simulink model "linear_vehicle_model"  (R2018a)
settings: Solver=VariableStepAuto  StartTime=0.0  StopTime=450  RelTol=1e-3
values from neighbouring files (symbols this model uses):
  Err_matrix = [1 -1 0 0 0 0 ... (first row only)    [Simulation_variables.m]
  vel_pos = [1 0 0]    [Simulation_variables.m]
  vel_vet = [0 1 0]    [Simulation_variables.m]
undefined symbols (not defined in the file or in its folder): controller, Reference, Vehicle, vehicleL
settings Model: Creator=um0002  LastModifiedBy=mw00361
settings SFSimCC: SimUseLocalCustomCode=on
settings RTWCC: RTWUseLocalCustomCode=on

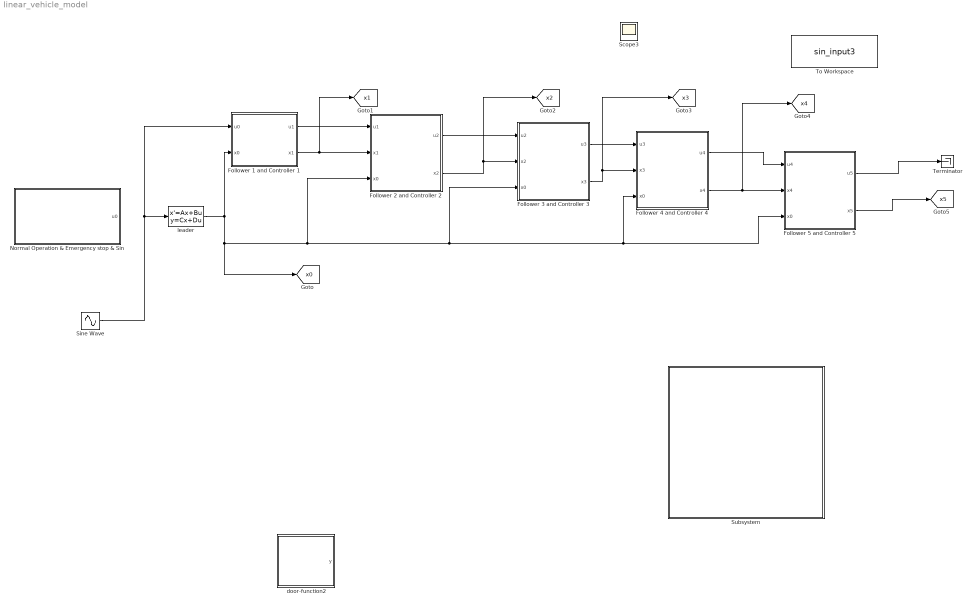
== system linear_vehicle_model ==
  Follower 1 and Controller 1 : Subsystem
  Follower 2 and Controller 2 : Subsystem
  Follower 3 and Controller 3 : Subsystem
  Follower 4 and Controller 4 : Subsystem
  Follower 5 and Controller 5 : Subsystem
  Normal Operation & Emergency stop & Sin : Subsystem
  Scope3 : Scope
  Sine Wave : Sin  Amplitude=200  Frequency=3  SampleTime=0
  Subsystem : Subsystem
  Terminator : Terminator
  To Workspace : ToWorkspace  VariableName=sin_input3  SaveFormat=Timeseries  SampleTime=-1
  door-function2 : Subsystem  mask{t_start=150, t_end=152, H=1.5}
      mask prompts: t_start "initial time"; t_end "final time"; H "height"
  leader : StateSpace  A=[0 1 0; 0 0 1; 0 0 -1/vehicleL.tau]  B=[0 0 1/vehicleL.tau]'  C=eye(3)  D=zeros(3,1)  InitialCondition=[100 75/3.6 0]'
  tag scope: x0=global, x1=global, x2=global, x3=global, x4=global, x5=global
  wires:
  Follower 1 and Controller 1/1("u1 ") -> Follower 2 and Controller 2/1(u1)
  Follower 1 and Controller 1/2(x1) -> [x1], Follower 2 and Controller 2/2(x1)
  Follower 2 and Controller 2/1("u2 ") -> Follower 3 and Controller 3/1(u2)
  Follower 3 and Controller 3/1("u3 ") -> Follower 4 and Controller 4/1(u3)
  Follower 3 and Controller 3/2(x3) -> [x3], Follower 4 and Controller 4/2(x3)
  Follower 2 and Controller 2/2(x2) -> [x2], Follower 3 and Controller 3/2(x2)
  leader/1 -> [x0], Follower 2 and Controller 2/3("x0 "), Follower 3 and Controller 3/3("x0 "), Follower 5 and Controller 5/3("x0 "), Follower 4 and Controller 4/3("x0 "), Follower 1 and Controller 1/2(x0)
  Follower 4 and Controller 4/1("u4 ") -> Follower 5 and Controller 5/1(u4)
  Follower 4 and Controller 4/2(x4) -> Follower 5 and Controller 5/2(x4), [x4]
  Follower 5 and Controller 5/1("u5 ") -> Terminator/1
  Follower 5 and Controller 5/2(x5) -> [x5]
  Sine Wave/1 -> Follower 1 and Controller 1/1(u0), leader/1

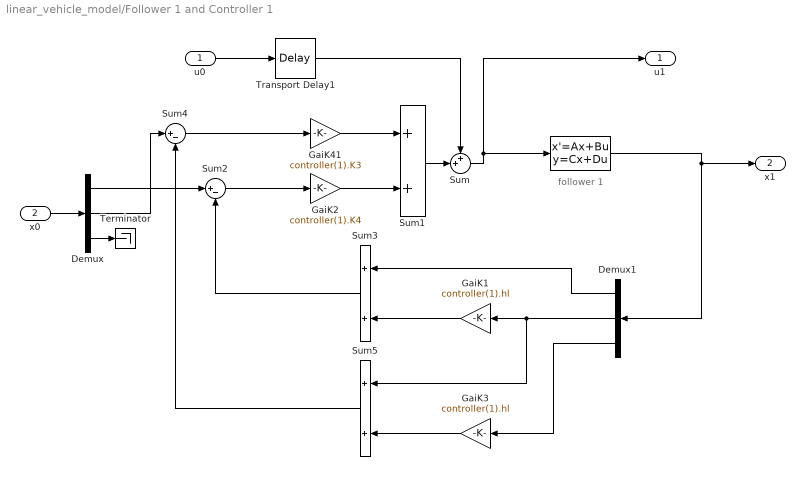
== system linear_vehicle_model/Follower 1 and Controller 1 ==
  note: follower 1
  u0 : Inport
  x0 : Inport  Port=2
  " " : StateSpace  A=[0 1 0; 0 0 1; 0 0 -1/vehicleL.tau]  B=[0 0 1/Vehicle(1).tau]'  C=eye(3)  D=zeros(3,1)  InitialCondition=[Vehicle(1).s0 75/3.6 0]'
  Demux : Demux  Outputs=3
  Demux1 : Demux  Outputs=3
  GaiK1 : Gain  Gain=controller(1).hl
  GaiK2 : Gain  Gain=controller(1).K4
  GaiK3 : Gain  Gain=controller(1).hl
  GaiK41 : Gain  Gain=controller(1).K3
  Sum : Sum  Inputs=++|
  Sum1 : Sum
  Sum2 : Sum  Inputs=|+-
  Sum3 : Sum
  Sum4 : Sum  Inputs=|+-
  Sum5 : Sum
  Terminator : Terminator
  Transport Delay1 : TransportDelay  DelayTime=Vehicle(1).delay
  "u1 " : Outport
  x1 : Outport  Port=2
  wires:
  " "/1 -> Demux1/1, x1/1
  u0/1 -> Transport Delay1/1
  x0/1 -> Demux/1
  Sum1/1 -> Sum/2
  Demux/1 -> Sum2/1
  Sum3/1 -> Sum2/2
  Demux1/1 -> Sum3/1
  Demux1/2 -> Sum5/1, GaiK1/1
  GaiK1/1 -> Sum3/2
  GaiK41/1 -> Sum1/1
  GaiK2/1 -> Sum1/2
  Sum2/1 -> GaiK2/1
  Demux/3 -> Terminator/1
  Sum4/1 -> GaiK41/1
  Demux/2 -> Sum4/1
  Demux1/3 -> GaiK3/1
  GaiK3/1 -> Sum5/2
  Sum5/1 -> Sum4/2
  Sum/1 -> " "/1, "u1 "/1
  Transport Delay1/1 -> Sum/1

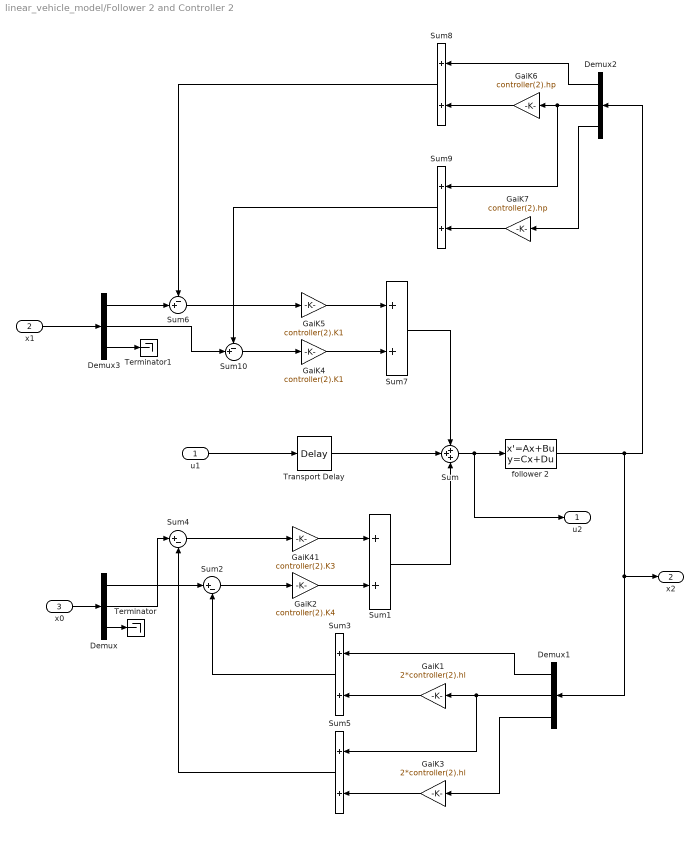
== system linear_vehicle_model/Follower 2 and Controller 2 ==
  u1 : Inport
  x1 : Inport  Port=2
  "x0 " : Inport  Port=3
  Demux{,1..3} (4 alike) : Demux  Outputs=3
  GaiK1 : Gain  Gain=2*controller(2).hl
  GaiK2 : Gain  Gain=controller(2).K4
  GaiK3 : Gain  Gain=2*controller(2).hl
  GaiK4 : Gain  Gain=controller(2).K1
  GaiK41 : Gain  Gain=controller(2).K3
  GaiK5 : Gain  Gain=controller(2).K1
  GaiK6 : Gain  Gain=controller(2).hp
  GaiK7 : Gain  Gain=controller(2).hp
  Sum : Sum  Inputs=+++
  Sum{1,3,5,7..9} (6 alike) : Sum
  Sum10 : Sum  Inputs=-+|
  Sum2 : Sum  Inputs=|+-
  Sum4 : Sum  Inputs=|+-
  Sum6 : Sum  Inputs=-+|
  Terminator : Terminator
  Terminator1 : Terminator
  Transport Delay : TransportDelay  DelayTime=Vehicle(1).delay
  follower 2 : StateSpace  A=[0 1 0; 0 0 1; 0 0 -1/vehicleL.tau]  B=[0 0 1/Vehicle(2).tau]'  C=eye(3)  D=zeros(3,1)  InitialCondition=[Vehicle(2).s0 75/3.6 0]'
  "u2 " : Outport
  x2 : Outport  Port=2
  wires:
  Sum5/1 -> Sum4/2
  GaiK3/1 -> Sum5/2
  Demux1/3 -> GaiK3/1
  Demux/2 -> Sum4/1
  Sum4/1 -> GaiK41/1
  Demux/3 -> Terminator/1
  Sum2/1 -> GaiK2/1
  GaiK2/1 -> Sum1/2
  GaiK41/1 -> Sum1/1
  GaiK1/1 -> Sum3/2
  Demux1/2 -> GaiK1/1, Sum5/1
  Demux1/1 -> Sum3/1
  Sum3/1 -> Sum2/2
  Demux/1 -> Sum2/1
  "x0 "/1 -> Demux/1
  Sum/1 -> follower 2/1, "u2 "/1
  follower 2/1 -> Demux2/1, x2/1, Demux1/1
  u1/1 -> Transport Delay/1
  x1/1 -> Demux3/1
  Demux3/3 -> Terminator1/1
  Sum7/1 -> Sum/1
  GaiK5/1 -> Sum7/1
  GaiK4/1 -> Sum7/2
  Demux2/1 -> Sum8/1
  Demux2/2 -> Sum9/1, GaiK6/1
  GaiK6/1 -> Sum8/2
  Demux3/1 -> Sum6/2
  Sum6/1 -> GaiK5/1
  Sum8/1 -> Sum6/1
  GaiK7/1 -> Sum9/2
  Demux2/3 -> GaiK7/1
  Sum10/1 -> GaiK4/1
  Demux3/2 -> Sum10/2
  Sum9/1 -> Sum10/1
  Transport Delay/1 -> Sum/2
  Sum1/1 -> Sum/3

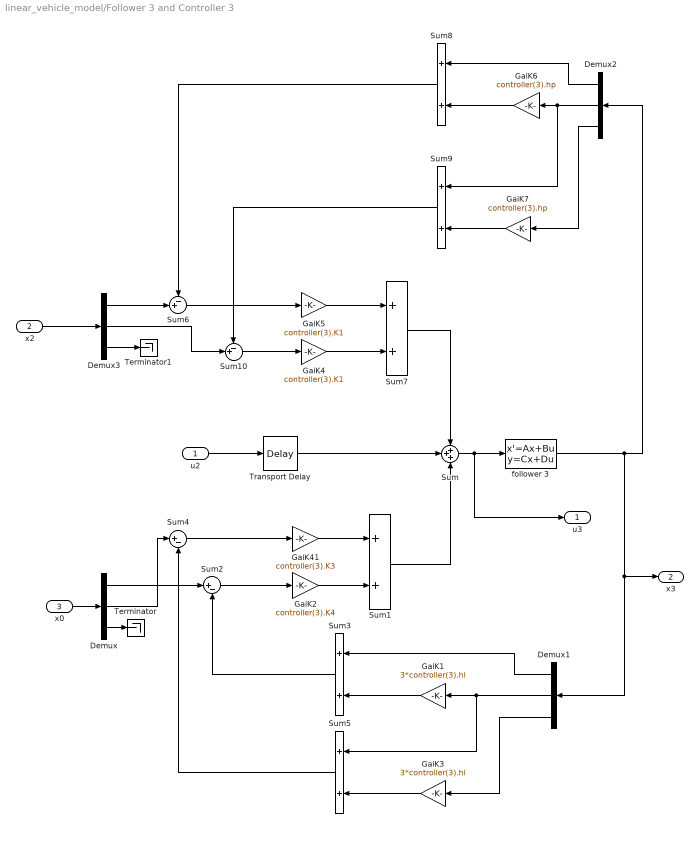
== system linear_vehicle_model/Follower 3 and Controller 3 ==
  u2 : Inport
  x2 : Inport  Port=2
  "x0 " : Inport  Port=3
  Demux{,1..3} (4 alike) : Demux  Outputs=3
  GaiK1 : Gain  Gain=3*controller(3).hl
  GaiK2 : Gain  Gain=controller(3).K4
  GaiK3 : Gain  Gain=3*controller(3).hl
  GaiK4 : Gain  Gain=controller(3).K1
  GaiK41 : Gain  Gain=controller(3).K3
  GaiK5 : Gain  Gain=controller(3).K1
  GaiK6 : Gain  Gain=controller(3).hp
  GaiK7 : Gain  Gain=controller(3).hp
  Sum : Sum  Inputs=+++
  Sum{1,3,5,7..9} (6 alike) : Sum
  Sum10 : Sum  Inputs=-+|
  Sum2 : Sum  Inputs=|+-
  Sum4 : Sum  Inputs=|+-
  Sum6 : Sum  Inputs=-+|
  Terminator : Terminator
  Terminator1 : Terminator
  Transport Delay : TransportDelay  DelayTime=Vehicle(1).delay
  follower 3 : StateSpace  A=[0 1 0; 0 0 1; 0 0 -1/vehicleL.tau]  B=[0 0 1/Vehicle(2).tau]'  C=eye(3)  D=zeros(3,1)  InitialCondition=[Vehicle(3).s0 75/3.6 0]'
  "u3 " : Outport
  x3 : Outport  Port=2
  wires:
  Sum9/1 -> Sum10/1
  Demux3/2 -> Sum10/2
  Sum10/1 -> GaiK4/1
  Demux2/3 -> GaiK7/1
  GaiK7/1 -> Sum9/2
  Sum8/1 -> Sum6/1
  Sum6/1 -> GaiK5/1
  Demux3/1 -> Sum6/2
  GaiK6/1 -> Sum8/2
  Demux2/2 -> GaiK6/1, Sum9/1
  Demux2/1 -> Sum8/1
  GaiK4/1 -> Sum7/2
  GaiK5/1 -> Sum7/1
  Sum7/1 -> Sum/1
  Demux3/3 -> Terminator1/1
  x2/1 -> Demux3/1
  u2/1 -> Transport Delay/1
  follower 3/1 -> Demux1/1, x3/1, Demux2/1
  Sum/1 -> follower 3/1, "u3 "/1
  "x0 "/1 -> Demux/1
  Demux/1 -> Sum2/1
  Sum3/1 -> Sum2/2
  Demux1/1 -> Sum3/1
  Demux1/2 -> Sum5/1, GaiK1/1
  GaiK1/1 -> Sum3/2
  GaiK41/1 -> Sum1/1
  GaiK2/1 -> Sum1/2
  Sum2/1 -> GaiK2/1
  Demux/3 -> Terminator/1
  Sum4/1 -> GaiK41/1
  Demux/2 -> Sum4/1
  Demux1/3 -> GaiK3/1
  GaiK3/1 -> Sum5/2
  Sum5/1 -> Sum4/2
  Transport Delay/1 -> Sum/2
  Sum1/1 -> Sum/3

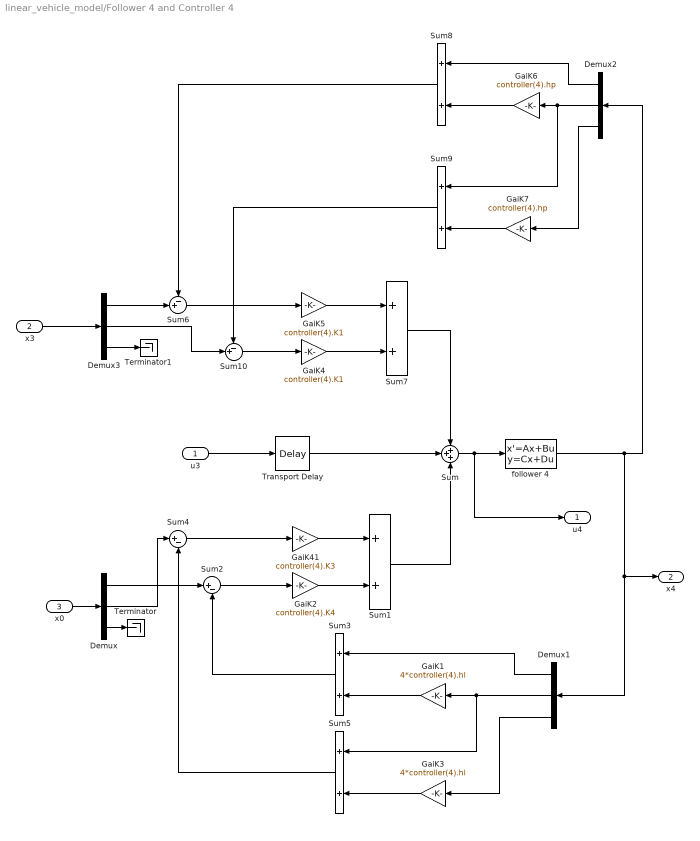
== system linear_vehicle_model/Follower 4 and Controller 4 ==
  u3 : Inport
  x3 : Inport  Port=2
  "x0 " : Inport  Port=3
  Demux{,1..3} (4 alike) : Demux  Outputs=3
  GaiK1 : Gain  Gain=4*controller(4).hl
  GaiK2 : Gain  Gain=controller(4).K4
  GaiK3 : Gain  Gain=4*controller(4).hl
  GaiK4 : Gain  Gain=controller(4).K1
  GaiK41 : Gain  Gain=controller(4).K3
  GaiK5 : Gain  Gain=controller(4).K1
  GaiK6 : Gain  Gain=controller(4).hp
  GaiK7 : Gain  Gain=controller(4).hp
  Sum : Sum  Inputs=+++
  Sum{1,3,5,7..9} (6 alike) : Sum
  Sum10 : Sum  Inputs=-+|
  Sum2 : Sum  Inputs=|+-
  Sum4 : Sum  Inputs=|+-
  Sum6 : Sum  Inputs=-+|
  Terminator : Terminator
  Terminator1 : Terminator
  Transport Delay : TransportDelay  DelayTime=Vehicle(1).delay
  follower 4 : StateSpace  A=[0 1 0; 0 0 1; 0 0 -1/vehicleL.tau]  B=[0 0 1/Vehicle(2).tau]'  C=eye(3)  D=zeros(3,1)  InitialCondition=[Vehicle(4).s0 75/3.6 0]'
  "u4 " : Outport
  x4 : Outport  Port=2
  wires:
  Sum5/1 -> Sum4/2
  GaiK3/1 -> Sum5/2
  Demux1/3 -> GaiK3/1
  Demux/2 -> Sum4/1
  Sum4/1 -> GaiK41/1
  Demux/3 -> Terminator/1
  Sum2/1 -> GaiK2/1
  GaiK2/1 -> Sum1/2
  GaiK41/1 -> Sum1/1
  GaiK1/1 -> Sum3/2
  Demux1/2 -> GaiK1/1, Sum5/1
  Demux1/1 -> Sum3/1
  Sum3/1 -> Sum2/2
  Demux/1 -> Sum2/1
  "x0 "/1 -> Demux/1
  Sum/1 -> follower 4/1, "u4 "/1
  follower 4/1 -> Demux2/1, x4/1, Demux1/1
  x3/1 -> Demux3/1
  Demux3/3 -> Terminator1/1
  Sum7/1 -> Sum/1
  GaiK5/1 -> Sum7/1
  GaiK4/1 -> Sum7/2
  Demux2/1 -> Sum8/1
  Demux2/2 -> Sum9/1, GaiK6/1
  GaiK6/1 -> Sum8/2
  Demux3/1 -> Sum6/2
  Sum6/1 -> GaiK5/1
  Sum8/1 -> Sum6/1
  GaiK7/1 -> Sum9/2
  Demux2/3 -> GaiK7/1
  Sum10/1 -> GaiK4/1
  Demux3/2 -> Sum10/2
  Sum9/1 -> Sum10/1
  u3/1 -> Transport Delay/1
  Transport Delay/1 -> Sum/2
  Sum1/1 -> Sum/3

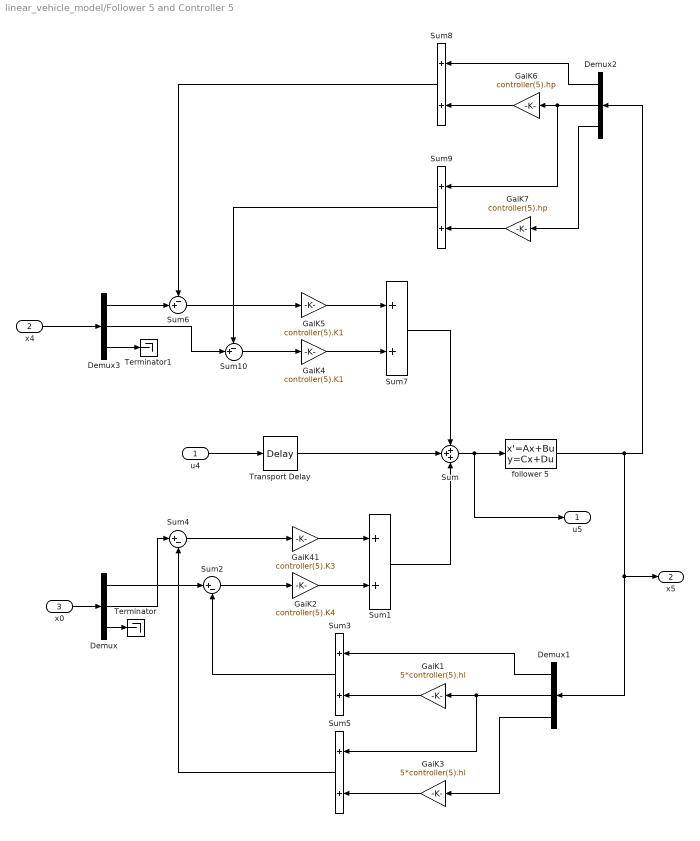
== system linear_vehicle_model/Follower 5 and Controller 5 ==
  u4 : Inport
  x4 : Inport  Port=2
  "x0 " : Inport  Port=3
  Demux{,1..3} (4 alike) : Demux  Outputs=3
  GaiK1 : Gain  Gain=5*controller(5).hl
  GaiK2 : Gain  Gain=controller(5).K4
  GaiK3 : Gain  Gain=5*controller(5).hl
  GaiK4 : Gain  Gain=controller(5).K1
  GaiK41 : Gain  Gain=controller(5).K3
  GaiK5 : Gain  Gain=controller(5).K1
  GaiK6 : Gain  Gain=controller(5).hp
  GaiK7 : Gain  Gain=controller(5).hp
  Sum : Sum  Inputs=+++
  Sum{1,3,5,7..9} (6 alike) : Sum
  Sum10 : Sum  Inputs=-+|
  Sum2 : Sum  Inputs=|+-
  Sum4 : Sum  Inputs=|+-
  Sum6 : Sum  Inputs=-+|
  Terminator : Terminator
  Terminator1 : Terminator
  Transport Delay : TransportDelay  DelayTime=Vehicle(1).delay
  follower 5 : StateSpace  A=[0 1 0; 0 0 1; 0 0 -1/vehicleL.tau]  B=[0 0 1/Vehicle(2).tau]'  C=eye(3)  D=zeros(3,1)  InitialCondition=[Vehicle(5).s0 75/3.6 0]'
  "u5 " : Outport
  x5 : Outport  Port=2
  wires:
  Sum5/1 -> Sum4/2
  GaiK3/1 -> Sum5/2
  Demux1/3 -> GaiK3/1
  Demux/2 -> Sum4/1
  Sum4/1 -> GaiK41/1
  Demux/3 -> Terminator/1
  Sum2/1 -> GaiK2/1
  GaiK2/1 -> Sum1/2
  GaiK41/1 -> Sum1/1
  GaiK1/1 -> Sum3/2
  Demux1/2 -> GaiK1/1, Sum5/1
  Demux1/1 -> Sum3/1
  Sum3/1 -> Sum2/2
  Demux/1 -> Sum2/1
  "x0 "/1 -> Demux/1
  Sum/1 -> follower 5/1, "u5 "/1
  follower 5/1 -> Demux2/1, x5/1, Demux1/1
  u4/1 -> Transport Delay/1
  x4/1 -> Demux3/1
  Demux3/3 -> Terminator1/1
  Sum7/1 -> Sum/1
  GaiK5/1 -> Sum7/1
  GaiK4/1 -> Sum7/2
  Demux2/1 -> Sum8/1
  Demux2/2 -> Sum9/1, GaiK6/1
  GaiK6/1 -> Sum8/2
  Demux3/1 -> Sum6/2
  Sum6/1 -> GaiK5/1
  Sum8/1 -> Sum6/1
  GaiK7/1 -> Sum9/2
  Demux2/3 -> GaiK7/1
  Sum10/1 -> GaiK4/1
  Demux3/2 -> Sum10/2
  Sum9/1 -> Sum10/1
  Transport Delay/1 -> Sum/2
  Sum1/1 -> Sum/3

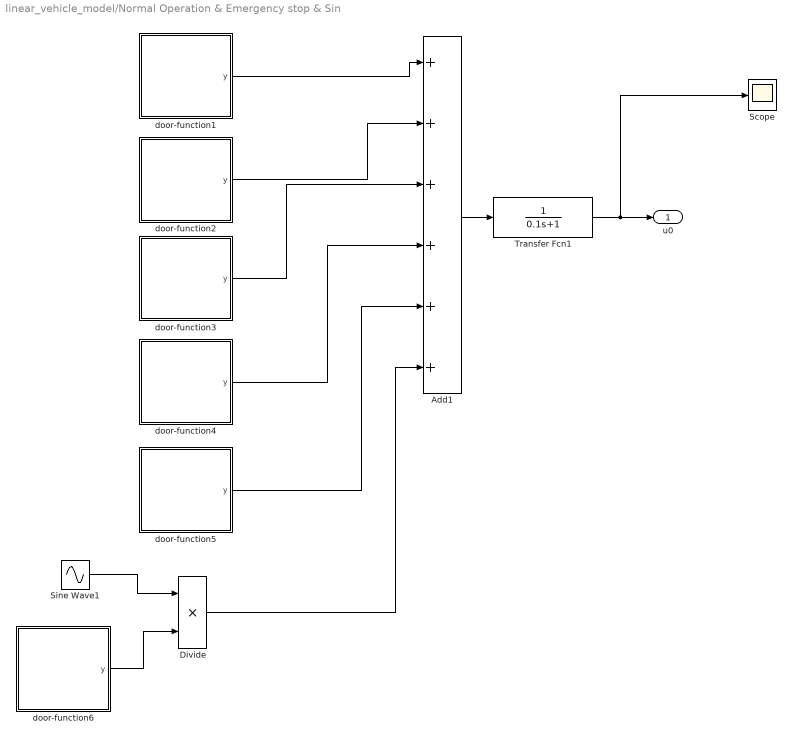
== system linear_vehicle_model/Normal Operation & Emergency stop & Sin ==
  Add1 : Sum  Inputs=++++++
  Divide : Product  Inputs=**
  Scope : Scope
  Sine Wave1 : Sin  Amplitude=0.6*9.81  Frequency=2*pi/15  SampleTime=0
  Transfer Fcn1 : TransferFcn  Denominator="[0.1  1]"
  door-function1 : Subsystem  mask{t_start=Reference.t_start(1), t_end=Reference.t_end(1), H=Reference.H(1)}
      mask prompts: t_start "initial time"; t_end "final time"; H "height"
  door-function2 : Subsystem  mask{t_start=Reference.t_start(2), t_end=Reference.t_end(2), H=Reference.H(2)}
      mask prompts: t_start "initial time"; t_end "final time"; H "height"
  door-function3 : Subsystem  mask{t_start=Reference.t_start(3), t_end=Reference.t_end(3), H=Reference.H(3)}
      mask prompts: t_start "initial time"; t_end "final time"; H "height"
  door-function4 : Subsystem  mask{t_start=Reference.t_start(4), t_end=Reference.t_end(4), H=Reference.H(4)}
      mask prompts: t_start "initial time"; t_end "final time"; H "height"
  door-function5 : Subsystem  mask{t_start=Reference.t_start(5), t_end=Reference.t_end(5), H=Reference.H(5)}
      mask prompts: t_start "initial time"; t_end "final time"; H "height"
  door-function6 : Subsystem  mask{t_start=Reference.t_start(6), t_end=Reference.t_end(6), H=Reference.H(6)}
      mask prompts: t_start "initial time"; t_end "final time"; H "height"
  u0 : Outport
  wires:
  Sine Wave1/1 -> Divide/1
  Transfer Fcn1/1 -> Scope/1, u0/1
  Add1/1 -> Transfer Fcn1/1
  door-function1/1(y) -> Add1/1
  door-function2/1(y) -> Add1/2
  door-function3/1(y) -> Add1/3
  door-function4/1(y) -> Add1/4
  door-function5/1(y) -> Add1/5
  door-function6/1(y) -> Divide/2
  Divide/1 -> Add1/6

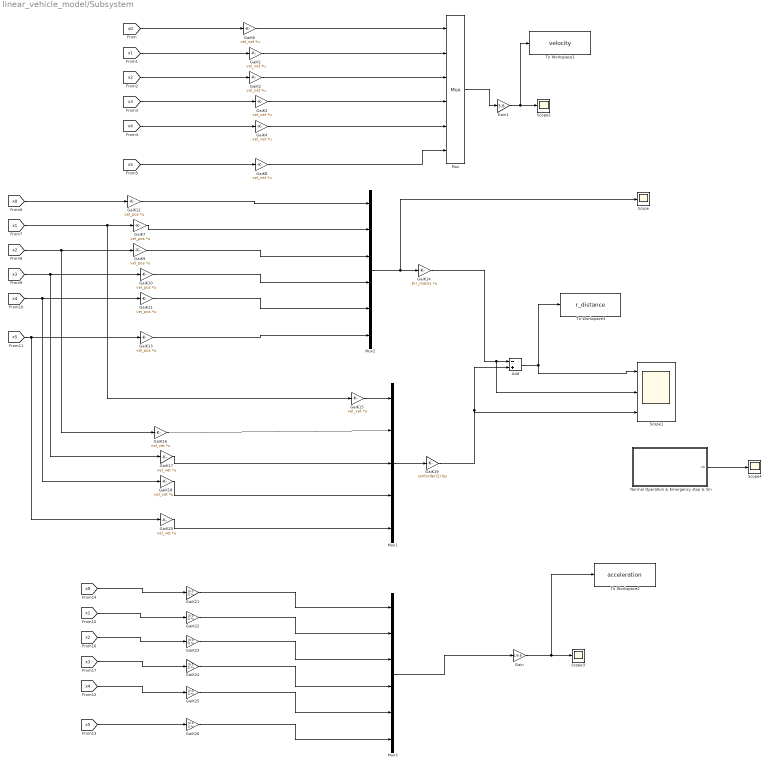
== system linear_vehicle_model/Subsystem ==
  Add : Sum  Inputs=-+
  GaiK{1..4,6,8,15..18,20} (11 alike) : Gain  Gain=vel_vet  Multiplication=Matrix(K*u)
  GaiK{7,9..13} (6 alike) : Gain  Gain=vel_pos  Multiplication=Matrix(K*u)
  GaiK14 : Gain  Gain=Err_matrix  Multiplication=Matrix(K*u)
  GaiK19 : Gain  Gain=controller(1).hp
  GaiK{21..26} (6 alike) : Gain  Gain=[0 0 1]  Multiplication=Matrix(K*u)
  Gain : Gain  Gain=1/9.8
  Gain1 : Gain  Gain=3.6
  Mux : Mux  Inputs=6
      settings: DisplayOption=signals
  Mux1 : Mux  Inputs=5
  Mux2 : Mux  Inputs=6
  Mux3 : Mux  Inputs=6
  Normal Operation & Emergency stop & Sin : Subsystem
  Scope{,2..4} (4 alike) : Scope
  Scope1 : Scope  NumInputPorts=3
  To Workspace1 : ToWorkspace  VariableName=velocity  SaveFormat=Timeseries  SampleTime=-1
  To Workspace2 : ToWorkspace  VariableName=acceleration  SaveFormat=Timeseries  SampleTime=-1
  To Workspace3 : ToWorkspace  VariableName=r_distance  SaveFormat=Timeseries  SampleTime=-1
  wires:
  GaiK2/1 -> Mux/3
  GaiK8/1 -> Mux/6
  GaiK6/1 -> Mux/1
  GaiK4/1 -> Mux/5
  GaiK1/1 -> Mux/2
  GaiK3/1 -> Mux/4
  [x4] -> GaiK4/1
  [x5] -> GaiK8/1
  [x0] -> GaiK6/1
  [x1] -> GaiK1/1
  [x2] -> GaiK2/1
  [x3] -> GaiK3/1
  [x0] -> GaiK12/1
  GaiK10/1 -> Mux2/4
  GaiK7/1 -> Mux2/2
  GaiK12/1 -> Mux2/1
  GaiK9/1 -> Mux2/3
  GaiK11/1 -> Mux2/5
  GaiK13/1 -> Mux2/6
  [x1] -> GaiK15/1, GaiK7/1
  [x5] -> GaiK20/1, GaiK13/1
  [x4] -> GaiK18/1, GaiK11/1
  [x3] -> GaiK17/1, GaiK10/1
  GaiK18/1 -> Mux1/4
  GaiK16/1 -> Mux1/2
  GaiK20/1 -> Mux1/5
  [x2] -> GaiK16/1, GaiK9/1
  GaiK15/1 -> Mux1/1
  GaiK17/1 -> Mux1/3
  GaiK14/1 -> Scope1/2, Add/1
  GaiK19/1 -> Scope1/3, Add/2
  Mux2/1 -> Scope/1, GaiK14/1
  Mux1/1 -> GaiK19/1
  Mux3/1 -> Gain/1
  [x0] -> GaiK21/1
  GaiK21/1 -> Mux3/1
  [x1] -> GaiK22/1
  GaiK22/1 -> Mux3/2
  [x2] -> GaiK23/1
  GaiK23/1 -> Mux3/3
  [x3] -> GaiK24/1
  GaiK24/1 -> Mux3/4
  [x4] -> GaiK25/1
  GaiK25/1 -> Mux3/5
  [x5] -> GaiK26/1
  GaiK26/1 -> Mux3/6
  Gain/1 -> To Workspace2/1, Scope3/1
  Mux/1 -> Gain1/1
  Add/1 -> Scope1/1, To Workspace3/1
  Normal Operation & Emergency stop & Sin/1(u0) -> Scope4/1
  Gain1/1 -> To Workspace1/1, Scope2/1

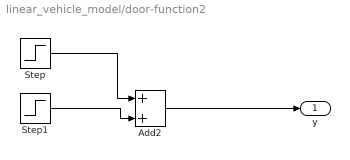
== system linear_vehicle_model/door-function2 ==
  Add2 : Sum
  Step : Step  Time=t_start  After=H  SampleTime=0
  Step1 : Step  Time=t_end  After=-H  SampleTime=0
  y : Outport
  wires:
  Add2/1 -> y/1
  Step1/1 -> Add2/2
  Step/1 -> Add2/1

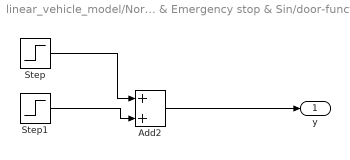
== system linear_vehicle_model/Normal Operation & Emergency stop & Sin/door-function1 ==
  Add2 : Sum
  Step : Step  Time=t_start  After=H  SampleTime=0
  Step1 : Step  Time=t_end  After=-H  SampleTime=0
  y : Outport
  wires:
  Step/1 -> Add2/1
  Step1/1 -> Add2/2
  Add2/1 -> y/1

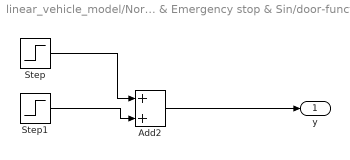
== system linear_vehicle_model/Normal Operation & Emergency stop & Sin/door-function2 ==
  Add2 : Sum
  Step : Step  Time=t_start  After=H  SampleTime=0
  Step1 : Step  Time=t_end  After=-H  SampleTime=0
  y : Outport
  wires:
  Add2/1 -> y/1
  Step1/1 -> Add2/2
  Step/1 -> Add2/1

== system linear_vehicle_model/Normal Operation & Emergency stop & Sin/door-function3 ==
  Add2 : Sum
  Step : Step  Time=t_start  After=H  SampleTime=0
  Step1 : Step  Time=t_end  After=-H  SampleTime=0
  y : Outport
  wires:
  Step/1 -> Add2/1
  Step1/1 -> Add2/2
  Add2/1 -> y/1

== system linear_vehicle_model/Normal Operation & Emergency stop & Sin/door-function4 ==
  Add2 : Sum
  Step : Step  Time=t_start  After=H  SampleTime=0
  Step1 : Step  Time=t_end  After=-H  SampleTime=0
  y : Outport
  wires:
  Add2/1 -> y/1
  Step1/1 -> Add2/2
  Step/1 -> Add2/1

== system linear_vehicle_model/Normal Operation & Emergency stop & Sin/door-function5 ==
  Add2 : Sum
  Step : Step  Time=t_start  After=H  SampleTime=0
  Step1 : Step  Time=t_end  After=-H  SampleTime=0
  y : Outport
  wires:
  Step/1 -> Add2/1
  Step1/1 -> Add2/2
  Add2/1 -> y/1

== system linear_vehicle_model/Normal Operation & Emergency stop & Sin/door-function6 ==
  Add2 : Sum
  Step : Step  Time=t_start  After=H  SampleTime=0
  Step1 : Step  Time=t_end  After=-H  SampleTime=0
  y : Outport
  wires:
  Add2/1 -> y/1
  Step1/1 -> Add2/2
  Step/1 -> Add2/1

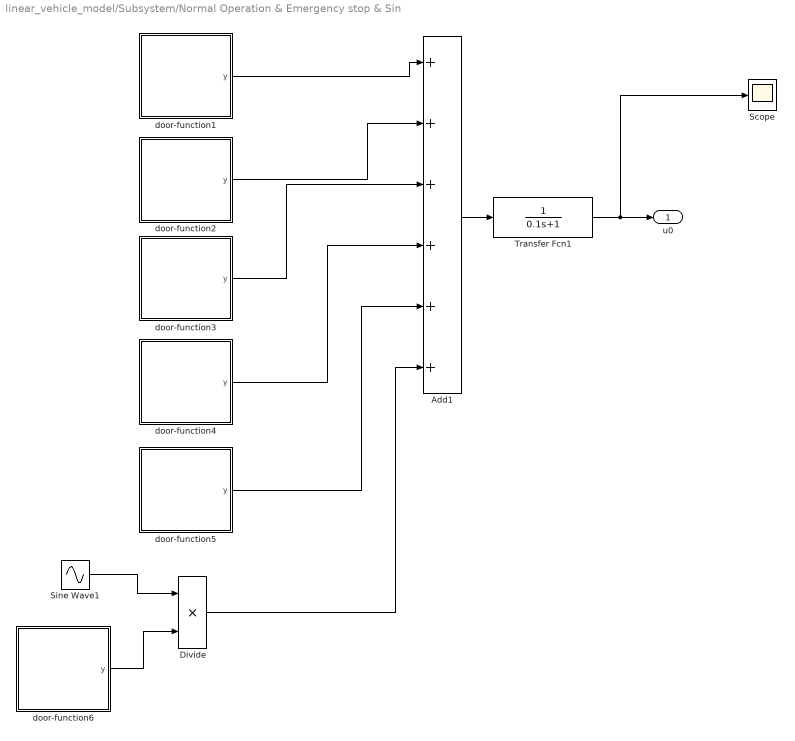
== system linear_vehicle_model/Subsystem/Normal Operation & Emergency stop & Sin ==
  Add1 : Sum  Inputs=++++++
  Divide : Product  Inputs=**
  Scope : Scope
  Sine Wave1 : Sin  Amplitude=0.6*9.81  Frequency=2*pi/15  SampleTime=0
  Transfer Fcn1 : TransferFcn  Denominator="[0.1  1]"
  door-function1 : Subsystem  mask{t_start=Reference.t_start(1), t_end=Reference.t_end(1), H=Reference.H(1)}
      mask prompts: t_start "initial time"; t_end "final time"; H "height"
  door-function2 : Subsystem  mask{t_start=Reference.t_start(2), t_end=Reference.t_end(2), H=Reference.H(2)}
      mask prompts: t_start "initial time"; t_end "final time"; H "height"
  door-function3 : Subsystem  mask{t_start=Reference.t_start(3), t_end=Reference.t_end(3), H=Reference.H(3)}
      mask prompts: t_start "initial time"; t_end "final time"; H "height"
  door-function4 : Subsystem  mask{t_start=Reference.t_start(4), t_end=Reference.t_end(4), H=Reference.H(4)}
      mask prompts: t_start "initial time"; t_end "final time"; H "height"
  door-function5 : Subsystem  mask{t_start=Reference.t_start(5), t_end=Reference.t_end(5), H=Reference.H(5)}
      mask prompts: t_start "initial time"; t_end "final time"; H "height"
  door-function6 : Subsystem  mask{t_start=Reference.t_start(6), t_end=Reference.t_end(6), H=Reference.H(6)}
      mask prompts: t_start "initial time"; t_end "final time"; H "height"
  u0 : Outport
  wires:
  Sine Wave1/1 -> Divide/1
  Transfer Fcn1/1 -> Scope/1, u0/1
  Add1/1 -> Transfer Fcn1/1
  door-function1/1(y) -> Add1/1
  door-function2/1(y) -> Add1/2
  door-function3/1(y) -> Add1/3
  door-function4/1(y) -> Add1/4
  door-function5/1(y) -> Add1/5
  door-function6/1(y) -> Divide/2
  Divide/1 -> Add1/6

== system linear_vehicle_model/Subsystem/Normal Operation & Emergency stop & Sin/door-function1 ==
  Add2 : Sum
  Step : Step  Time=t_start  After=H  SampleTime=0
  Step1 : Step  Time=t_end  After=-H  SampleTime=0
  y : Outport
  wires:
  Step/1 -> Add2/1
  Step1/1 -> Add2/2
  Add2/1 -> y/1

== system linear_vehicle_model/Subsystem/Normal Operation & Emergency stop & Sin/door-function2 ==
  Add2 : Sum
  Step : Step  Time=t_start  After=H  SampleTime=0
  Step1 : Step  Time=t_end  After=-H  SampleTime=0
  y : Outport
  wires:
  Add2/1 -> y/1
  Step1/1 -> Add2/2
  Step/1 -> Add2/1

== system linear_vehicle_model/Subsystem/Normal Operation & Emergency stop & Sin/door-function3 ==
  Add2 : Sum
  Step : Step  Time=t_start  After=H  SampleTime=0
  Step1 : Step  Time=t_end  After=-H  SampleTime=0
  y : Outport
  wires:
  Step/1 -> Add2/1
  Step1/1 -> Add2/2
  Add2/1 -> y/1

== system linear_vehicle_model/Subsystem/Normal Operation & Emergency stop & Sin/door-function4 ==
  Add2 : Sum
  Step : Step  Time=t_start  After=H  SampleTime=0
  Step1 : Step  Time=t_end  After=-H  SampleTime=0
  y : Outport
  wires:
  Add2/1 -> y/1
  Step1/1 -> Add2/2
  Step/1 -> Add2/1

== system linear_vehicle_model/Subsystem/Normal Operation & Emergency stop & Sin/door-function5 ==
  Add2 : Sum
  Step : Step  Time=t_start  After=H  SampleTime=0
  Step1 : Step  Time=t_end  After=-H  SampleTime=0
  y : Outport
  wires:
  Step/1 -> Add2/1
  Step1/1 -> Add2/2
  Add2/1 -> y/1

== system linear_vehicle_model/Subsystem/Normal Operation & Emergency stop & Sin/door-function6 ==
  Add2 : Sum
  Step : Step  Time=t_start  After=H  SampleTime=0
  Step1 : Step  Time=t_end  After=-H  SampleTime=0
  y : Outport
  wires:
  Add2/1 -> y/1
  Step1/1 -> Add2/2
  Step/1 -> Add2/1
